simulink model "board_specific_NUCLEO_F446_CANsend"  (R2016b)
settings: Solver=FixedStepDiscrete  StartTime=0.0  StopTime=10.0  FixedStep=1e-3  RelTol=1e-3
libraries: mbed_lib x7
settings Model: Creator=EW  LastModifiedBy=oh
settings DataIOCC: LimitDataPoints=on  SaveFormat=Array
settings OptimizationCC: LifeSpan=1
settings DebuggingCC: SFUnexpectedBacktrackingDiag=warning  SFNoUnconditionalDefaultTransitionDiag=warning  SFExecutionAtInitializationDiag=none
settings HardwareCC: ProdBitPerPointer=32  ProdBitPerSizeT=32  ProdBitPerPtrDiffT=32  ProdLargestAtomicInteger=Long  ProdLargestAtomicFloat=Double  ProdIntDivRoundTo=Undefined  ProdWordSize=32  ProdHWDeviceType=ARM Compatible->ARM Cortex
settings ModelReferenceCC: PropagateSignalLabelsOutOfModel=off
settings RTWCC: SystemTargetFile=mbed.tlc  TemplateMakefile=mbed.tmf  Description=Mbed Target (Embedded Target)  TargetLang=C++
settings CodeAppCC: IgnoreCustomStorageClasses=off
settings STFCustomTargetCC: TargetLibSuffix=.a  GenerateSampleERTMain=on  CombineOutputUpdateFcns=on  ERTCustomFileBanners=on  SupportContinuousTime=off  SupportNonInlinedSFcns=off  RemoveResetFunc=on  MATLABClassNameForMDSCustomization=Simulink.SoftwareTarget.ERTCustomization  GRTInterface=off  SystemTargetFile=mbed.tlc
settings ERTTargetCC: GenerateSampleERTMain=on  ParMdlRefBuildCompliant=off  CompOptLevelCompliant=off  ConcurrentExecutionCompliant=off  ERTFirstTimeCompliant=off  ModelStepFunctionPrototypeControlCompliant=off  CPPClassGenCompliant=off  UseToolchainInfoCompliant=off  ERTCustomFileTemplate=mbed_file_process.tlc  ConvertIfToSwitch=off  SuppressUnreachableDefaultCases=off
settings ConfigComp: CovMetricSettings=dw  CovHtmlReporting=on  CovSaveCumulativeToWorkspaceVar=on  CovSaveSingleToWorkspaceVar=on  CovExternalEMLEnable=off

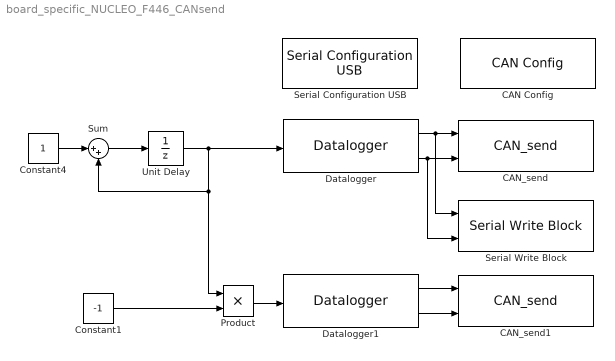
== system board_specific_NUCLEO_F446_CANsend ==
  CAN Config : mbed_lib/Serial/CAN/CAN Config  CAN_ID=1  CAN_Tx_Port=A  CAN_Tx_Pin=12  CAN_Rx_Port=A  CAN_Rx_Pin=11  CAN_frequency=1000000
  CAN_send : mbed_lib/Serial/CAN/CAN_send  Priority=11  CAN_ID=1  Msg_ID=10  SampleTime=-1
  CAN_send1 : mbed_lib/Serial/CAN/CAN_send  Priority=10  CAN_ID=1  Msg_ID=20  SampleTime=-1
  Constant1 : Constant  Value=-1  OutDataTypeStr=int16  SampleTime=0.5
  Constant4 : Constant  OutDataTypeStr=uint16  SampleTime=1
  Datalogger : mbed_lib/Utilities/Datalogger  TypeInputPorts={ 'uint16' 1 }  TypeOfInputs={'1*uint16'}  BufferSize=100  errEn=off  SampleTime=-1
  Datalogger1 : mbed_lib/Utilities/Datalogger  TypeInputPorts={ 'int16' 1 }  TypeOfInputs={'1*int16'}  BufferSize=100  errEn=off  SampleTime=-1
  Product : Product  OutDataTypeStr=int16
  Serial Configuration USB : mbed_lib/Serial/UART/Serial Configuration USB  BaudRate=9600
  Serial Write Block : mbed_lib/Serial/UART/Serial Write Block  SerialPort=0  numData=on  SampleTime=-1
  Sum : Sum  Inputs=|++
  Unit Delay : UnitDelay  SampleTime=-1
  wires:
  Unit Delay/1 -> Datalogger/1, Product/1, Sum/2
  Datalogger/2 -> Serial Write Block/2, CAN_send/2
  Datalogger/1 -> Serial Write Block/1, CAN_send/1
  Constant4/1 -> Sum/1
  Sum/1 -> Unit Delay/1
  Datalogger1/1 -> CAN_send1/1
  Datalogger1/2 -> CAN_send1/2
  Product/1 -> Datalogger1/1
  Constant1/1 -> Product/2
